simulink model "model_ensemble_two_hydro_DVPP"  (R2020a)
settings: Solver=ode15s  StartTime=0.0  StopTime=200  MaxStep=1/60  RelTol=1e-2  AbsTol=1e-1  EnableMultiTasking=on
PreLoadFcn:
  | %load_Nordic32_data;
values from neighbouring files (symbols this model uses):
  Fbat = tf(0)    [main_ensemble_two_hydro_DVPP.m]
  fn = 50    [load_data_ensemble_two_hydro_DVPP.m]
  K_ideal = R*(1+6.5*s)/((1+2*s)*(1+17*s))    [main_ensemble_two_hydro_DVPP.m]
  Pgen = [40;  40 ; 80*100]    [load_data_ensemble_two_hydro_DVPP.m]
  POPT = min(POPT,MBASE)    [load_data_ensemble_two_hydro_DVPP.m]
  Pwind0 = POPT(1)    [main_ensemble_two_hydro_DVPP.m]
  time_activate_wind = 40    [load_data_ensemble_two_hydro_DVPP.m]
  time_event = 45    [load_data_ensemble_two_hydro_DVPP.m]
  wind_turbines = table(BUS,BSKV,MBASE,POPT,V_WIND,ROT_OPT, ROT_RATED)    [load_data_ensemble_two_hydro_DVPP.m]
undefined symbols (not defined in the file or in its folder): FCR
libraries: Nordic32_Lib x11, powerlib x3
settings Model: Creator=Innocent  LastModifiedBy=joakbj
settings SolverCC: AutoScaleAbsTol=off  MaxOrder=2  ZeroCrossAlgorithm=Adaptive
settings DataIOCC: SaveFormat=Array  SaveOutput=off  SaveTime=off  ReturnWorkspaceOutputs=off
settings OptimizationCC: BlockReduction=off  BooleanDataType=off  ExpressionDepthLimit=2147483647  InitFltsAndDblsToZero=on  LifeSpan=inf
settings DebuggingCC: AlgebraicLoopMsg=none  SaveWithParameterizedLinksMsg=none  UnderspecifiedInitializationDetection=Classic  MergeDetectMultiDrivingBlocksExec=none  SignalResolutionControl=TryResolveAllWithWarning  IgnoredZcDiagnostic=none  MultiTaskDSMMsg=warning  MultiTaskCondExecSysMsg=none  FcnCallInpInsideContextMsg=warning  UnconnectedInputMsg=none  UnconnectedOutputMsg=none  UnconnectedLineMsg=none  StateNameClashWarn=warning  StrictBusMsg=ErrorOnBusTreatedAsVector  SFUnexpectedBacktrackingDiag=warning  SFNoUnconditionalDefaultTransitionDiag=warning  SFExecutionAtInitializationDiag=none  ArithmeticOperatorsInVariantConditions=warning
settings HardwareCC: ProdBitPerPointer=32  ProdBitPerSizeT=32  ProdBitPerPtrDiffT=32  ProdLargestAtomicFloat=None  ProdIntDivRoundTo=Undefined  ProdEndianess=Unspecified  ProdWordSize=32  ProdHWDeviceType=32-bit Generic
settings ModelReferenceCC: PropagateSignalLabelsOutOfModel=off
settings SFSimCC: SimUseLocalCustomCode=off  CustomCodeUndefinedFunction=UseInterfaceOnly
settings RTWCC: RTWUseLocalCustomCode=off
settings CodeAppCC: StateflowObjectComments=on
settings GRTTargetCC: TargetFcnLib=ansi_tfl_tmw.mat  TargetLangStandard=C89/C90 (ANSI)  CombineOutputUpdateFcns=off  GRTInterface=on
settings ConfigComp: CovMetricSettings=dw  CovHtmlReporting=on  CovSaveCumulativeToWorkspaceVar=on  CovSaveSingleToWorkspaceVar=on  CovExternalEMLEnable=off
settings SimscapeCC: SimscapeNormalizeSystem=off

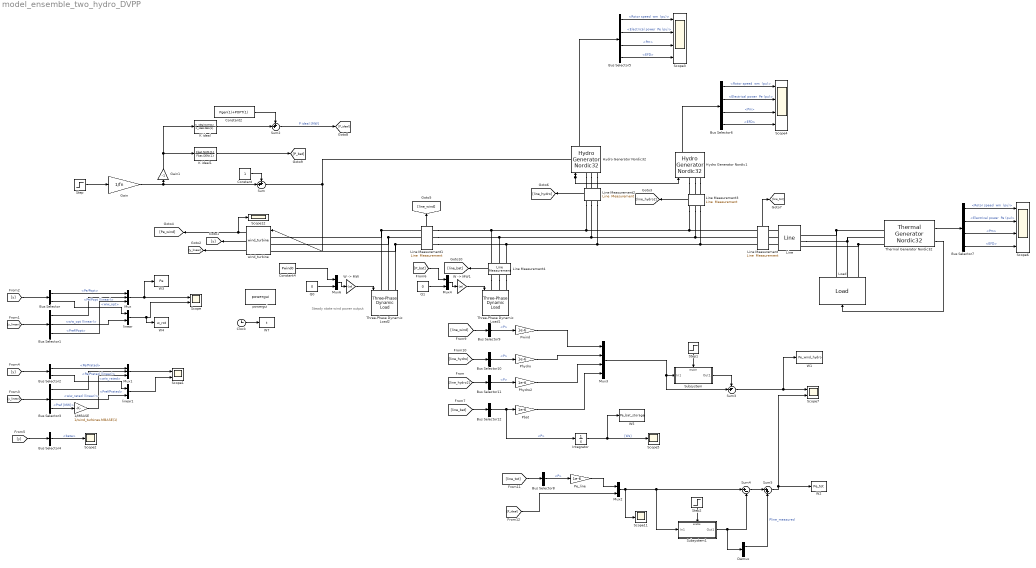
== system model_ensemble_two_hydro_DVPP ==
  note: Steady state wind power output
  1/MBASE : Gain  Gain=1/wind_turbines.MBASE(1)
  Bus Selector : BusSelector  OutputSignals=Pe/Popt,w/w_opt
  Bus Selector1 : BusSelector  OutputSignals=Pe/Popt (linear),w/w_opt (linear),Pref/Popt
  Bus Selector{8..12} (5 alike) : BusSelector  OutputSignals=P
  Bus Selector2 : BusSelector  OutputSignals=Pe/Prated,w/w_rated
  Bus Selector3 : BusSelector  OutputSignals=Pe/Prated (linear),w/w_rated (linear),Pref [MW]
  Bus Selector4 : BusSelector  OutputSignals=beta
  Bus Selector5 : BusSelector  OutputSignals="Rotor speed  wm  (pu),Electrical power  Pe (pu),Pm,EFD"
  Bus Selector6 : BusSelector  OutputSignals="Rotor speed  wm  (pu),Electrical power  Pe (pu),Pm,EFD"
  Bus Selector7 : BusSelector  OutputSignals="Rotor speed  wm  (pu),Electrical power  Pe (pu),Pm,EFD"
  Clock : Clock
  Constant : Constant
  Constant2 : Constant  Value=Pgen(1)+POPT(1)
  Constant4 : Constant  Value=Pwind0
  Demux : Demux  Outputs=2
  Gain : Gain  Gain=1/fn
  Gain1 : Gain  Gain=-1
  Hydro Generator Nordic1 : Nordic32_Lib/Hydro Generator Nordic32  i=2  gen_data=GenData  pss_data=PSSData  exc_data=ExcData  ii=2  FCR_reg=FCR{2}  fn=fn  open_loop_on=1
      link override Generator: InitialConditions=[0 -58.7141 0.807148 0.807148 0.807148 -8.27698 -128.277 111.723 1.49129]
      link override Pref: Value=0.8
      link override Turbine & Regulators/Excitation/Excitation Standard: v0=[1 1.4913]
      link override Turbine & Regulators/Hydraulic Turbine and Governor_modified: po=0.8
      link override Vref: Value=1
  Hydro Generator Nordic32 : Nordic32_Lib/Hydro Generator Nordic32  i=1  gen_data=GenData  pss_data=PSSData  exc_data=ExcData  ii=1  FCR_reg=FCR{1}  fn=fn  open_loop_on=1
      link override Generator: InitialConditions=[0 -58.7141 0.807148 0.807148 0.807148 -8.27698 -128.277 111.723 1.49129]
      link override Pref: Value=0.8
      link override Turbine & Regulators/Excitation/Excitation Standard: v0=[1 1.4913]
      link override Turbine & Regulators/Hydraulic Turbine and Governor_modified: po=0.8
      link override Vref: Value=1
  Integrator : Integrator
  K ideal : TransferFcn  Numerator=K_ideal.NUM{1}  Denominator=K_ideal.DEN{1}
  K ideal1 : TransferFcn  Numerator=Fbat.NUM{1}  Denominator=Fbat.DEN{1}
  Line : Nordic32_Lib/Line  i=1  data=lines  fn=fn
      link override Distributed Parameters Line: x1=[1.75766174168727e-08 396589.116227462 396590.020292506;314.159265358979 314.159265358979 314.159265358979;1.11754234374664 0.89322943618934 -0.677570867843288]  x2=[1.84695909701856e-08 396434.682277798 396435.591263281;314.159265358979 314.159265358979 314.159265358979;1.0783094486618 0.890263482532115 -0.680536814780748]  x3=[3.97601517592064e-11 1262.79466175231 1262.79802838049;314.159265358979 314.159265358979 314.159265358979;-0.656279460329388 0.8948270041266 -0.675973996187751]  x4=[4.21692753469767e-11 1664.84662440988 1664.84992963874;314.159265358979 314.159265358979 314.159265358979;1.89136505659244 0.870352209998365 -0.700447567218935]  x5=0.000113108313399149
  Line Measurement{,1..4} (5 alike) : Nordic32_Lib/Line  Measurement  SystemSampleTime=-1  Latency=0  AutoFrameSizeCalculation=off
      settings: PortSchema="{\"entries\":[{\"content\":{\"sides\":[{\"content\":{\"connectorIds\":[\"LConn1\",\"LConn2\",\"LConn3\"]},\"type\":\"ConnectorPlacement.EquallySpacedRectSide\",\"uuid\":\"159cc543-018e-4826-b622-a4d07c97e386\"},{\"content\":{\"connectorIds\":[\"RConn1\",\"RConn2\",\"RConn3\"],\"side\":\"RIGHT\"},\"type\":\"ConnectorPlacement.EquallySpacedRectSide\",\"uuid\":\"cb1aeae8-69bb-45ac-8689-4e8674d58501\"},{\"content\":{\"connectorIds\":[\"Out1\"],\"side\":\"TOP\"},\"type\":\"ConnectorPlacement.EquallySpacedRectSide\",\"uuid\":\"62a962af-3de7-4ff9-a859-7af1186eef9e\"}]},\"type\":\"ConnectorPlacement.EquallySpacedConnector\",\"uuid\":\"81b99b7d-1491-4204-9648-8ec0c780f157\"}],\"packageUris\":[\"http://schema.mathworks.com/mf0/Connector/19700101\"],\"version\":\"1.0\"}"
  Load : Nordic32_Lib/Load  i=2  data=loads  fn=fn
      link override Three-Phase Dynamic Load: ActiveReactivePowers=[0 0]  PositiveSequence=[0.991087 22.2497]
      link override Three-Phase Parallel C Load: NominalVoltage=(400000)*0.991087
  Mux : Mux  Inputs=3
  Mux1 : Mux  Inputs=3
  Mux2 : Mux  Inputs=2
  Mux3 : Mux
  Mux4 : Mux  Inputs=2
  Mux6 : Mux  Inputs=2
  Pbat : Gain  Gain=1e-6
  Pe_line : Gain  Gain=1e-6
  Phydro : Gain  Gain=1e-6
  Phydro2 : Gain  Gain=1e-6
  Pwind : Gain  Gain=1e-6
  Q0 : Constant  Value=0
  Q1 : Constant  Value=0
  Scope : Scope  NumInputPorts=2
  Scope1 : Scope  NumInputPorts=2
  Scope{2,5,11..12} (4 alike) : Scope
  Scope3 : Scope  NumInputPorts=4
  Scope4 : Scope  NumInputPorts=4
  Scope6 : Scope  NumInputPorts=4
  Scope7 : Scope  NumInputPorts=2
  Step : Step  Time=time_event  After=-1  SampleTime=0
  Step1 : Step  Time=time_activate_wind+1  Before=1  After=0  SampleTime=0
  Step2 : Step  Time=time_activate_wind+1  Before=1  After=0  SampleTime=0
  Subsystem : Subsystem
  Subsystem1 : Subsystem
  Sum : Sum  Inputs=++|
  Sum2 : Sum  Inputs=++|
  Sum3 : Sum  Inputs=-+|
  Sum4 : Sum  Inputs=|+-
  Sum5 : Sum  Inputs=|++
  Thermal Generator Nordic32 : Nordic32_Lib/Thermal Generator Nordic32  i=3  gen_data=GenData  pss_data=PSSData  exc_data=ExcData  fn=fn
      link override Generator: BusType=swing  InitialConditions=[0 -33.3121 0.901288 0.901288 0.901288 -7.76423 -127.764 112.236 2.46014]
      link override Pref: Value=0.89303
      link override Turbine & Regulators/Excitation/Excitation Standard: v0=[1 2.4601]
      link override Vref: Value=1
  Three-Phase Dynamic Load1 : powerlib/Elements/Three-Phase Dynamic Load  NominalVoltage=[ 400*1e3 fn ]  ActiveReactivePowers=[0 0]  PositiveSequence=[0.991473 22.4197]  ExternalControl=on  NpNq=[1.3 2]  TimeConstants="[0  0  0  0]"  MinimumVoltage=0.7  Tfilter=1e-4  LoadFlowParameters=[4,0,0,0,0]
      settings: SourceProductBaseCode=PS
  Three-Phase Dynamic Load2 : powerlib/Elements/Three-Phase Dynamic Load  NominalVoltage=[ 400*1e3 fn ]  ActiveReactivePowers=[0 0]  PositiveSequence=[0.991473 22.4197]  ExternalControl=on  NpNq=[1.3 2]  TimeConstants="[0  0  0  0]"  MinimumVoltage=0.7  Tfilter=1e-4  LoadFlowParameters=[4,0,0,0,0]
      settings: SourceProductBaseCode=PS
  "W -> MW" : Gain  Gain=-1e6
  "W -> MW1" : Gain  Gain=-1e6
  W1 : ToWorkspace  VariableName=Pe_wind_hydro  SampleTime=1/60
  W2 : ToWorkspace  VariableName=Pe_tot  SampleTime=1/60
  W3 : ToWorkspace  VariableName=Pe  SampleTime=1/60
  W4 : ToWorkspace  VariableName=w_rot  SampleTime=1/60
  W5 : ToWorkspace  VariableName=Pe_bat_storage  SampleTime=1/60
  W7 : ToWorkspace  VariableName=t  SampleTime=1/60
  linear : Mux  Inputs=2
  linear1 : Mux  Inputs=2
  powergui : powerlib/powergui  Priority=2  SimulationMode=Phasor  SampleTime=0  frequency=50  Iterations=100  frequencyindice=50  Pbase=100e6  ErrMax=1e-06  UnitsV=kV  UnitsW=MW  buscounter=3  FunctionMessages=off  echomessages=off  EnableUseOfTLC=off  CurrentSourceSwitches=off  DisableSnubberDevices=off  DisableRonSwitches=off  DisableVfSwitches=off  DisplayEquations=off  AutomaticDiscreteSolvers=off  SolverType=Tustin/Backward Euler (TBE)  Interpol=off  ExternalGateDelay=off  methode=off  Ts=100  x0status=blocks  SPID=off  SwTol=0  HookPort=off  NonlinearTolerance=1e-4  nMaxIteration=100  ContinueOnMaxIteration=off  RestoreLinks=warning  ResistiveCurrentMeasurement=off  Frange=logspace(0,3,50)  Ylog=off  Xlog=off  ShowGrid=off  save=off  variable=ZData  structure=0  ZoomFFT=on  StartTime=0.0  cycles=1  DisplayStyle=1  fundamental=60  FreqAxis=off  MaxFrequency=1000  frequencyindicesteady=1  RmsSteady=1  display=off
  wind_turbine : Nordic32_Lib/wind_turbine  i=1  data=wind_turbines  data_NREL=data_NREL  fn=fn  time_activate_wind=time_activate_wind  Gwind=Gwind  Gwind_speed=Gwind_speed  FCR=FCR{3}
      link override Three-Phase Dynamic Load2: ActiveReactivePowers=[0 0]  PositiveSequence=[0.991473 22.4197]
  wires:
  Clock/1 -> W7/1
  wind_turbine/2 -> [y]
  wind_turbine/3 -> [y_linear]
  [y] -> Bus Selector/1
  [y_linear] -> Bus Selector1/1
  Bus Selector/1 -> Mux/1  "<Pe/Popt>"
  Bus Selector1/1 -> Mux/2  "<Pe/Popt (linear)>"
  Bus Selector1/3 -> Mux/3  "<Pref/Popt>"
  Bus Selector/2 -> linear/1  "<w/w_opt>"
  Bus Selector1/2 -> linear/2  "<w/w_opt (linear)>"
  Mux/1 -> W3/1, Scope/1
  linear/1 -> W4/1, Scope/2
  linear1/1 -> Scope1/2
  Bus Selector3/2 -> linear1/2  "<w/w_rated (linear)>"
  Bus Selector3/3 -> 1/MBASE/1  "<Pref [MW]>"
  Bus Selector3/1 -> Mux1/2  "<Pe/Prated (linear)>"
  Mux1/1 -> Scope1/1
  [y] -> Bus Selector2/1
  Bus Selector2/2 -> linear1/1  "<w/w_rated>"
  [y_linear] -> Bus Selector3/1
  Bus Selector2/1 -> Mux1/1  "<Pe/Prated>"
  1/MBASE/1 -> Mux1/3  "<Pref/Prated>"
  [y] -> Bus Selector4/1
  Bus Selector4/1 -> Scope2/1  "<beta>"
  Thermal Generator Nordic32/2 -> Load/1
  Bus Selector7/4 -> Scope6/4  "<EFD>"
  Bus Selector7/2 -> Scope6/2  "<Electrical power  Pe (pu)>"
  Thermal Generator Nordic32/1 -> Bus Selector7/1
  Bus Selector7/3 -> Scope6/3  "<Pm>"
  Bus Selector7/1 -> Scope6/1  "<Rotor speed  wm  (pu)>"
  Step/1 -> Gain/1
  Constant/1 -> Sum/1
  Gain/1 -> Sum/2, Gain1/1
  Gain1/1 -> K ideal1/1, K ideal/1
  K ideal/1 -> Sum2/2
  Sum2/1 -> [P_ideal]  "P ideal [MW]"
  wind_turbine/1 -> [Pe_wind], Scope12/1
  Constant2/1 -> Sum2/1
  Sum/1 -> wind_turbine/1, Hydro Generator Nordic1/1, Hydro Generator Nordic32/1
  Bus Selector9/1 -> Pwind/1  "<P>"
  Line Measurement1/1 -> [line_wind]
  [line_wind] -> Bus Selector9/1
  Q0/1 -> Mux6/2
  "W -> MW"/1 -> Three-Phase Dynamic Load2/1
  Mux6/1 -> "W -> MW"/1
  Constant4/1 -> Mux6/1
  Line Measurement2/1 -> [line_hydro]
  [line_hydro] -> Bus Selector10/1
  Bus Selector10/1 -> Phydro/1  "<P>"
  Line Measurement/1 -> [line_tot]
  [line_tot] -> Bus Selector8/1
  Bus Selector8/1 -> Pe_line/1  "<P>"
  Pwind/1 -> Mux3/1
  Phydro/1 -> Mux3/2
  Pe_line/1 -> Mux2/1
  [P_ideal] -> Mux2/2
  Mux2/1 -> Scope11/1, Subsystem1/1(In1), Sum4/1
  Step1/1 -> Subsystem/Enable
  Mux3/1 -> Sum3/2, Subsystem/1(In1)
  Subsystem/1(Out1) -> Sum3/1
  Sum3/1 -> W1/1, Scope7/1
  Step2/1 -> Subsystem1/Enable
  Subsystem1/1(Out1) -> Demux/1, Sum4/2
  Sum5/1 -> W2/1, Scope7/2
  Sum4/1 -> Sum5/1
  Demux/1 -> Sum5/2  "Pline_measured"
  Bus Selector5/4 -> Scope3/4  "<EFD>"
  Hydro Generator Nordic32/1 -> Bus Selector5/1
  Bus Selector5/1 -> Scope3/1  "<Rotor speed  wm  (pu)>"
  Bus Selector5/3 -> Scope3/3  "<Pm>"
  Bus Selector5/2 -> Scope3/2  "<Electrical power  Pe (pu)>"
  Bus Selector6/2 -> Scope4/2  "<Electrical power  Pe (pu)>"
  Bus Selector6/3 -> Scope4/3  "<Pm>"
  Hydro Generator Nordic1/1 -> Bus Selector6/1
  Line Measurement3/1 -> [line_hydro2]
  Bus Selector6/4 -> Scope4/4  "<EFD>"
  Bus Selector6/1 -> Scope4/1  "<Rotor speed  wm  (pu)>"
  [line_hydro2] -> Bus Selector11/1
  Bus Selector11/1 -> Phydro2/1  "<P>"
  Phydro2/1 -> Mux3/3
  K ideal1/1 -> [P_bat]
  Line Measurement4/1 -> [line_bat]
  [P_bat] -> Mux4/1
  "W -> MW1"/1 -> Three-Phase Dynamic Load1/1
  Q1/1 -> Mux4/2
  Mux4/1 -> "W -> MW1"/1
  [line_bat] -> Bus Selector12/1
  Bus Selector12/1 -> Integrator/1, Pbat/1  "<P>"
  Pbat/1 -> Mux3/4
  Integrator/1 -> W5/1, Scope5/1  "[Ws]"
  connections:
  Line Measurement1/RConn1 -- Line Measurement4/RConn1 -- Line Measurement2/RConn1 -- Line Measurement3/RConn1 -- Line Measurement/LConn1
  Line Measurement1/RConn2 -- Line Measurement4/RConn2 -- Line Measurement2/RConn2 -- Line Measurement3/RConn2 -- Line Measurement/LConn2
  Line Measurement1/RConn3 -- Line Measurement4/RConn3 -- Line Measurement2/RConn3 -- Line Measurement3/RConn3 -- Line Measurement/LConn3
  Thermal Generator Nordic32/LConn1 -- Load/RConn1 -- Line/RConn1
  Line/RConn2 -- Thermal Generator Nordic32/LConn2 -- Load/RConn2
  Thermal Generator Nordic32/LConn3 -- Load/RConn3 -- Line/RConn3
  Line/LConn1 -- Line Measurement/RConn1
  Line/LConn2 -- Line Measurement/RConn2
  Line/LConn3 -- Line Measurement/RConn3
  Line Measurement1/LConn1 -- Three-Phase Dynamic Load2/LConn1 -- wind_turbine/LConn1
  Line Measurement1/LConn2 -- Three-Phase Dynamic Load2/LConn2 -- wind_turbine/LConn2
  Line Measurement1/LConn3 -- Three-Phase Dynamic Load2/LConn3 -- wind_turbine/LConn3
  Hydro Generator Nordic32/LConn1 -- Line Measurement2/LConn1
  Hydro Generator Nordic32/LConn2 -- Line Measurement2/LConn2
  Hydro Generator Nordic32/LConn3 -- Line Measurement2/LConn3
  Hydro Generator Nordic1/LConn2 -- Line Measurement3/LConn2
  Hydro Generator Nordic1/LConn3 -- Line Measurement3/LConn3
  Hydro Generator Nordic1/LConn1 -- Line Measurement3/LConn1
  Line Measurement4/LConn1 -- Three-Phase Dynamic Load1/LConn1
  Line Measurement4/LConn2 -- Three-Phase Dynamic Load1/LConn2
  Line Measurement4/LConn3 -- Three-Phase Dynamic Load1/LConn3

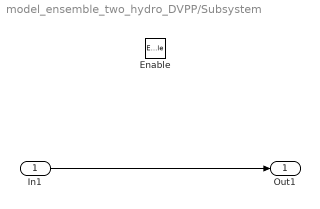
== system model_ensemble_two_hydro_DVPP/Subsystem ==
  In1 : Inport
  Enable : EnablePort
  Out1 : Outport
  wires:
  In1/1 -> Out1/1

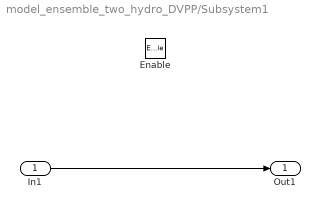
== system model_ensemble_two_hydro_DVPP/Subsystem1 ==
  In1 : Inport
  Enable : EnablePort
  Out1 : Outport
  wires:
  In1/1 -> Out1/1
